simulink model "AUAV_V3_TestSensors"  (R2015a)
settings: Solver=FixedStepDiscrete  StartTime=0.0  StopTime=10.0  FixedStep=T  RelTol=1e-3
PreLoadFcn:
  | %T = 0.0025;
  | MavlinkBus;
  | mcuInit;
  | % Baro Altitude Computation
  | % =========================
  | basePressure = 98192.64;
  | baseTemp = 288.215;
  | lapseRate = -0.00198122;
  | baseHeight = 0;
values from neighbouring files (symbols this model uses):
  apSampleTime = 0.01    [mcuInit.m]
  latlong_WP = 1    [mcuInit.m]
  mavlink_attitude_t = Simulink.Bus    [MavlinkBusMarcello.m]
  mavlink_gps_raw_int_t = Simulink.Bus    [MavlinkBus.m]    (also in MavlinkBusMarcello.m)
  mavlink_raw_imu_t = Simulink.Bus    [MavlinkBus.m]    (also in MavlinkBusMarcello.m)
  mavlink_scaled_pressure_t = Simulink.Bus    [MavlinkBus.m]    (also in MavlinkBusMarcello.m)
  mavlink_servo_output_raw_t = Simulink.Bus    [MavlinkBusMarcello.m]
  mavlink_slugs_navigation_t = Simulink.Bus    [MavlinkBusMarcello.m]
  mavlink_sys_status_t = Simulink.Bus    [MavlinkBus.m]    (also in MavlinkBusMarcello.m)
  T = 0.01    [mcuInit.m]
  Xpoints = [0 0]    [mcuInit.m]
  Ypoints = [0 0]    [mcuInit.m]
  Zpoints = [0 0]    [mcuInit.m]
undefined symbols (not defined in the file or in its folder): A0, A14, A15, A2, A3, A4, A5, A6, accBiasRateLimit, B0, bankCommandLimit, barAdjust, baroCutoff, baroCutTemp, cubeAccelGain16405, cubeGyroGain16405, cubeMagGain16405, D0, D11, D7, D8, daLimit, data, daTrimMax, daTrimMin, deLimit, deTrimMax, deTrimMin, drLimit, drTrimMax, drTrimMin, dtLimit, dtTrimMax, dtTrimMin, F2, F3, G0, G13, G15, gaind, GS_location, gyroBiasRateLimit, IC1max, IPStar, ISA_g, Max, maxAcc, MaxDwnPthStar, maxDynPressure, maxEta, mlParamInterface, ms, OC1max, P112, P125, P127, P16, P20, P21, P30 ... (+26)
undefined symbols (not defined in the file): baroOffset, baroScale, barTGain1, barTGain2, barTMean1, barTMean2, bda, bde, bdr, bdt, bICda, bICde, bICdr, bICdt, derivativesConstant, lowRateSensorCutoff, mainSensorCutoff, mda, mde, mdr, mdt, mICda, mICde, mICdr, mICdt, pitotOffset, pitotScale, pitTGain1, pitTGain2, pitTMean1, pitTMean2, powerOffset, powerScale, pressureSensorCutoff, tempOffset, tempScale, vzCutoff, xCutoff, yCutoff
libraries: MCHP_Blockset x158, simulink x84, SLUGS_Library x31, aerolibconvert2 x6, aerolibutil x4, aerolibtransform2 x3, dspmtrx3 x2, aerolibobsolete x2
(part 13 of 24)

== system AUAV_V3_TestSensors/Inner Loop// Navigation/L1 Output Feedback Controller With Projection Operator/Trapezoidal Integrator ==
  x : Inport
  Reset : Inport  Port=2
  Constant : Constant  Value=1/3  OutDataTypeStr=single
  Constant1 : Constant  Value=4/3  OutDataTypeStr=single
  Constant2 : Constant  Value=T/2  OutDataTypeStr=single
  Constant3 : Constant  Value=1/3  OutDataTypeStr=single
  Constant5 : Constant  Value=0  OutDataTypeStr=single
  Integer Delay : Delay  DelayLength=1  InputProcessing=Inherited  SampleTime=T
  Integer Delay1 : Delay  InputProcessing=Inherited  SampleTime=T
  Integer Delay2 : Delay  DelayLength=1  InputProcessing=Inherited  SampleTime=T
  Product{,1..3} (4 alike) : Product  OutDataTypeStr=single  RndMeth=Zero
  Protect NaNs : Subsystem
  Protect NaNs1 : Subsystem
  Subtract : Sum  Inputs=3  OutDataTypeStr=single
  Subtract1 : Sum  Inputs=2  OutDataTypeStr=single
  Switch1 : Switch  Criteria=u2 > Threshold  Threshold=0.3  SampleTime=.01
  "[min max]" : Saturate  UpperLimit=upperLimit  LowerLimit=lowerLimit  SampleTime=T
  Int(x) : Outport
  wires:
  Constant/1 -> Product/2
  Constant1/1 -> Product1/2
  Integer Delay/1 -> Product1/1
  Integer Delay1/1 -> Product2/1
  Constant3/1 -> Product2/2
  x/1 -> Protect NaNs/1(In1)
  Product/1 -> Subtract/1
  Product1/1 -> Subtract/2
  Product2/1 -> Subtract/3
  Constant2/1 -> Product3/1
  Subtract/1 -> Product3/2
  Integer Delay2/1 -> Subtract1/1
  Constant5/1 -> Switch1/1
  Reset/1 -> Switch1/2
  Switch1/1 -> Protect NaNs1/1(In1)
  "[min max]"/1 -> Switch1/3
  Product3/1 -> Subtract1/2
  Subtract1/1 -> "[min max]"/1
  Protect NaNs/1(Out1) -> Product/1, Integer Delay/1, Integer Delay1/1
  Protect NaNs1/1(Out1) -> Int(x)/1, Integer Delay2/1

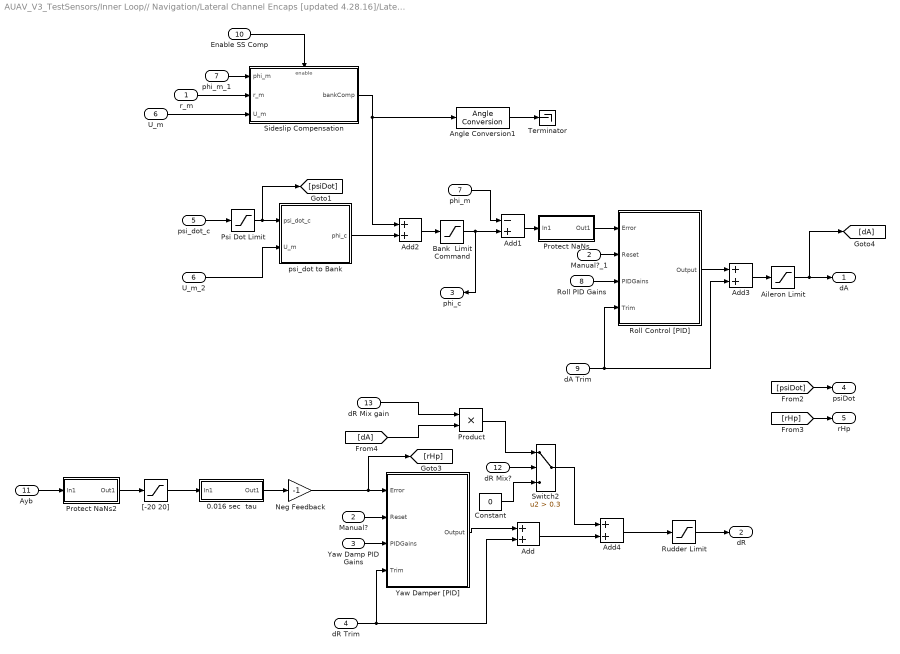
== system AUAV_V3_TestSensors/Inner Loop// Navigation/Lateral Channel Encaps [updated 4.28.16]/Lateral Channel ==
  r_m : Inport
  Manual? : Inport  Port=2
  Yaw Damp PID Gains : Inport  Port=3
  dR Trim : Inport  Port=4
  psi_dot_c : Inport  Port=5
  U_m : Inport  Port=6
  phi_m : Inport  Port=7
  Roll PID Gains : Inport  Port=8
  dA Trim : Inport  Port=9
  Enable SS Comp : Inport  Port=10
  Ayb : Inport  Port=11
  dR Mix? : Inport  Port=12
  dR Mix gain : Inport  Port=13
  0.016 sec  tau : Subsystem  mask(Tustin1stOrderLowpassAutoInitialCondition){f=10, T=T}
      mask prompts: f "Lowpass Frequency"; T "Sample Time"
      mask help: Takes a 3db rolloff frequency (in Hz, NOT radians/s) and a sample time. Performs a symbolic Tustin conversion and implements in a discrete filter. The initial output of the filter is set by the first sample.
      mask Help: Enter the desired 3db rolloff frequency in Hz and the sample time. Initial conditions are sampled automatically.
      mask Display: fprintf('%.2f Hz lowpass',f)
  Add{,2..4} (4 alike) : Sum  OutDataTypeStr=single
  Add1 : Sum  Inputs=-+  OutDataTypeStr=single
  Aileron Limit : Saturate  UpperLimit=daLimit  LowerLimit=-daLimit  SampleTime=apSampleTime
  Angle Conversion1 : aerolibconvert2/Angle Conversion  IU=rad  OU=deg
  Bank  Limit Command : Saturate  UpperLimit=bankCommandLimit  LowerLimit=-bankCommandLimit  SampleTime=apSampleTime
  Constant : Constant  Value=0  OutDataTypeStr=single
  Manual?_1 : InportShadow  Port=2
  "Neg Feedback " : Gain  Gain=-1  OutDataTypeStr=float('single')
  Product : Product  RndMeth=Zero
  Protect NaNs : Subsystem
  Protect NaNs2 : Subsystem
  Psi Dot Limit : Saturate  UpperLimit=1  LowerLimit=-1  SampleTime=apSampleTime
  Roll Control [PID] : Subsystem  AncestorBlock=SLUGS_Library/Control Blocks/PID Controller w//Anti-Windup  mask(PID){Tsample=apSampleTime, Ndelay=derivativesConstant, upperSaturationLimit=daLimit, lowerSaturationLimit=-daLimit}
      mask prompts: Tsample "Sample Time"; Ndelay "Integer delays for de/dt"; upperSaturationLimit "Upper Saturation Limit"; lowerSaturationLimit "Lower Saturation Limit"
      mask help: PID controller block with anti-windup and saturation limits. Implemented as a discrete forwardl integration which stops integrating when the output is saturated. Derivative is implemented as a numerical derivative with N integer delays to smooth output.
      mask Display:
      | disp('PID')
      | port_label('input',1,'error')
      | port_label('input',3,'gains')
      | port_label('input',2,'reset')
      | port_label('input',4,'trim')
      | port_label('output',1,'output')
  Rudder Limit : Saturate  UpperLimit=drLimit  LowerLimit=-drLimit  SampleTime=apSampleTime
  Sideslip Compensation : Subsystem
  Switch2 : Switch  Criteria=u2 > Threshold  Threshold=0.3  InputSameDT=on
  Terminator : Terminator
  U_m_2 : InportShadow  Port=6
  Yaw Damper [PID] : Subsystem  AncestorBlock=SLUGS_Library/Control Blocks/PID Controller w//Anti-Windup  mask(PID){Tsample=apSampleTime, Ndelay=derivativesConstant, upperSaturationLimit=drLimit, lowerSaturationLimit=-drLimit}
      mask prompts: Tsample "Sample Time"; Ndelay "Integer delays for de/dt"; upperSaturationLimit "Upper Saturation Limit"; lowerSaturationLimit "Lower Saturation Limit"
      mask help: PID controller block with anti-windup and saturation limits. Implemented as a discrete forwardl integration which stops integrating when the output is saturated. Derivative is implemented as a numerical derivative with N integer delays to smooth output.
      mask Display:
      | disp('PID')
      | port_label('input',1,'error')
      | port_label('input',3,'gains')
      | port_label('input',2,'reset')
      | port_label('input',4,'trim')
      | port_label('output',1,'output')
  "[-20 20]" : Saturate  UpperLimit=20  LowerLimit=-20
  phi_m_1 : InportShadow  Port=7
  psi_dot to Bank : Subsystem  AncestorBlock=SLUGS_Library/Navigation/psi_dot to Bank
  dA : Outport
  dR : Outport  Port=2
  phi_c : Outport  Port=3
  psiDot : Outport  Port=4
  rHp : Outport  Port=5
  wires:
  [rHp] -> rHp/1
  [psiDot] -> psiDot/1
  [dA] -> Product/2
  dR Mix gain/1 -> Product/1
  Product/1 -> Switch2/1
  Constant/1 -> Switch2/3
  dR Mix?/1 -> Switch2/2
  Switch2/1 -> Add4/1
  Add/1 -> Add4/2
  Add4/1 -> Rudder Limit/1
  Angle Conversion1/1 -> Terminator/1
  "[-20 20]"/1 -> 0.016 sec  tau/1(In1)
  Protect NaNs2/1(Out1) -> "[-20 20]"/1
  Protect NaNs/1(Out1) -> Roll Control [PID]/1(Error)
  Rudder Limit/1 -> dR/1
  0.016 sec  tau/1(Out1) -> "Neg Feedback "/1
  "Neg Feedback "/1 -> Yaw Damper [PID]/1(Error), [rHp]
  Ayb/1 -> Protect NaNs2/1(In1)
  Enable SS Comp/1 -> Sideslip Compensation/Enable
  U_m/1 -> Sideslip Compensation/3(U_m)
  r_m/1 -> Sideslip Compensation/2(r_m)
  phi_m_1/1 -> Sideslip Compensation/1(phi_m)
  Sideslip Compensation/1(bankComp) -> Angle Conversion1/1, Add2/1
  psi_dot to Bank/1(phi_c) -> Add2/2
  Add2/1 -> Bank  Limit Command/1
  U_m_2/1 -> psi_dot to Bank/2(U_m)
  Manual?/1 -> Yaw Damper [PID]/2(Reset)
  Yaw Damp PID Gains/1 -> Yaw Damper [PID]/3(PIDGains)
  Yaw Damper [PID]/1(Output) -> Add/1
  dR Trim/1 -> Yaw Damper [PID]/4(Trim), Add/2
  Manual?_1/1 -> Roll Control [PID]/2(Reset)
  Roll PID Gains/1 -> Roll Control [PID]/3(PIDGains)
  Add3/1 -> Aileron Limit/1
  Roll Control [PID]/1(Output) -> Add3/1
  dA Trim/1 -> Roll Control [PID]/4(Trim), Add3/2
  Aileron Limit/1 -> [dA], dA/1
  Add1/1 -> Protect NaNs/1(In1)
  phi_m/1 -> Add1/1
  Bank  Limit Command/1 -> phi_c/1, Add1/2
  Psi Dot Limit/1 -> [psiDot], psi_dot to Bank/1(psi_dot_c)
  psi_dot_c/1 -> Psi Dot Limit/1

== system AUAV_V3_TestSensors/Inner Loop// Navigation/Lateral Channel Encaps [updated 4.28.16]/psi_dot_c Select logic1 ==
  psi_dot_ad : Inport
  L1OnOff : Inport  Port=2
  psi_dot_c_noNav : Inport  Port=3
  IsPassThrough : Inport  Port=4
  nav_phi_c : Inport  Port=5
  U_m : Inport  Port=6
  Bank to Psi Dot : Subsystem  AncestorBlock=SLUGS_Library/Navigation/Bank to Psi Dot
  Switch : Switch  Criteria=u2 > Threshold  Threshold=0.3
  Switch1 : Switch  Criteria=u2 > Threshold  Threshold=0.3  InputSameDT=on
  psi_dot_c : Outport
  psi_dot_c_4_L1 : Outport  Port=2
  wires:
  U_m/1 -> Bank to Psi Dot/2(U_m)
  nav_phi_c/1 -> Bank to Psi Dot/1(phi_c)
  IsPassThrough/1 -> Switch1/2
  psi_dot_c_noNav/1 -> Switch1/1
  Switch/1 -> psi_dot_c/1
  L1OnOff/1 -> Switch/2
  psi_dot_ad/1 -> Switch/1
  Switch1/1 -> psi_dot_c_4_L1/1, Switch/3
  Bank to Psi Dot/1(psi_dot_c) -> Switch1/3

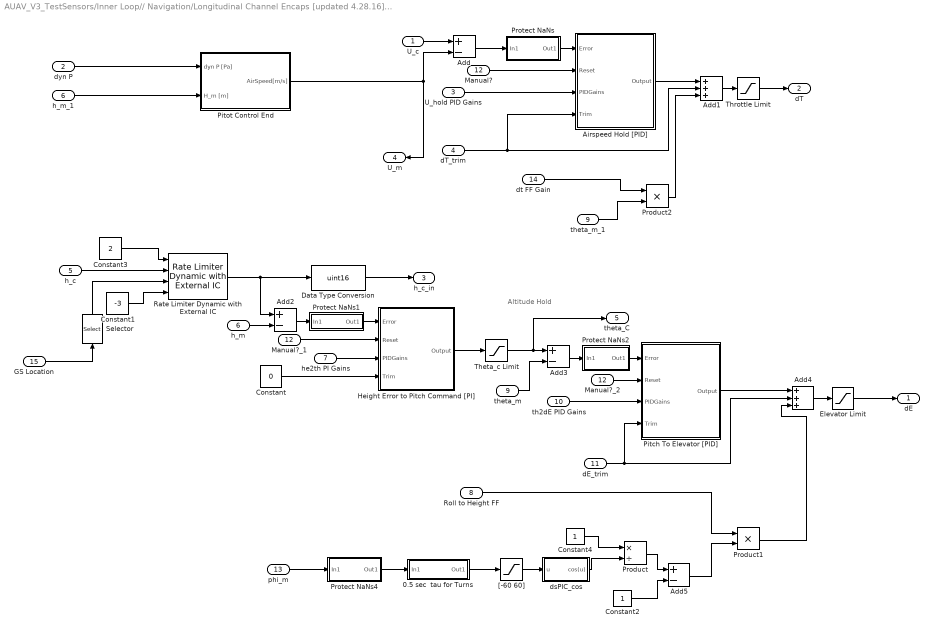
== system AUAV_V3_TestSensors/Inner Loop// Navigation/Longitudinal Channel Encaps [updated 4.28.16]/Longitudinal Channel ==
  note: Altitude Hold
  U_c : Inport
  dyn P : Inport  Port=2
  U_hold PID Gains : Inport  Port=3
  dT_trim : Inport  Port=4
  h_c : Inport  Port=5
  h_m : Inport  Port=6
  he2th PI Gains : Inport  Port=7
  Roll to Height FF : Inport  Port=8
  theta_m : Inport  Port=9
  th2dE PID Gains : Inport  Port=10
  dE_trim : Inport  Port=11
  Manual? : Inport  Port=12
  phi_m : Inport  Port=13
  dt FF Gain : Inport  Port=14
  GS Location : Inport  Port=15
  0.5 sec  tau for Turns : Subsystem  mask(Tustin1stOrderLowpassAutoInitialCondition){f=0.32, T=T}
      mask prompts: f "Lowpass Frequency"; T "Sample Time"
      mask help: Takes a 3db rolloff frequency (in Hz, NOT radians/s) and a sample time. Performs a symbolic Tustin conversion and implements in a discrete filter. The initial output of the filter is set by the first sample.
      mask Help: Enter the desired 3db rolloff frequency in Hz and the sample time. Initial conditions are sampled automatically.
      mask Display: fprintf('%.2f Hz lowpass',f)
  Add : Sum  Inputs=+-
  Add1 : Sum  Inputs=3  OutDataTypeStr=single
  Add2 : Sum  Inputs=+-  OutDataTypeStr=single
  Add3 : Sum  Inputs=+-  OutDataTypeStr=single
  Add4 : Sum  Inputs=3  OutDataTypeStr=single
  Add5 : Sum  Inputs=+-  OutDataTypeStr=single
  Airspeed Hold [PID] : Subsystem  AncestorBlock=SLUGS_Library/Control Blocks/PID Controller w//Anti-Windup  mask(PID){Tsample=apSampleTime, Ndelay=derivativesConstant, upperSaturationLimit=dtLimit, lowerSaturationLimit=0}
      mask prompts: Tsample "Sample Time"; Ndelay "Integer delays for de/dt"; upperSaturationLimit "Upper Saturation Limit"; lowerSaturationLimit "Lower Saturation Limit"
      mask help: PID controller block with anti-windup and saturation limits. Implemented as a discrete forwardl integration which stops integrating when the output is saturated. Derivative is implemented as a numerical derivative with N integer delays to smooth output.
      mask Display:
      | disp('PID')
      | port_label('input',1,'error')
      | port_label('input',3,'gains')
      | port_label('input',2,'reset')
      | port_label('input',4,'trim')
      | port_label('output',1,'output')
  Constant : Constant  Value=0
  Constant1 : Constant  Value=-3  OutDataTypeStr=single
  Constant2 : Constant  OutDataTypeStr=single
  Constant3 : Constant  Value=2  OutDataTypeStr=single
  Constant4 : Constant  OutDataTypeStr=single
  Data Type Conversion : DataTypeConversion  OutDataTypeStr=uint16
  Elevator Limit : Saturate  UpperLimit=deLimit  LowerLimit=-deLimit  SampleTime=apSampleTime
  Height Error to Pitch Command [PI] : Subsystem  AncestorBlock=SLUGS_Library/Control Blocks/PI Controller w//Anti-Windup  mask(PID){Tsample=apSampleTime, Ndelay=derivativesConstant, upperSaturationLimit=pitchCommandLimit, lowerSaturationLimit=-pitchCommandLimit}
      mask prompts: Tsample "Sample Time"; Ndelay "Integer delays for de/dt"; upperSaturationLimit "Upper Saturation Limit"; lowerSaturationLimit "Lower Saturation Limit"
      mask help: PID controller block with anti-windup and saturation limits. Implemented as a discrete forwardl integration which stops integrating when the output is saturated. Derivative is implemented as a numerical derivative with N integer delays to smooth output.
      mask Display:
      | disp('PI')
      | port_label('input',1,'error')
      | port_label('input',3,'gains')
      | port_label('input',2,'reset')
      | port_label('input',4,'trim')
      | port_label('output',1,'output')
  Manual?_1 : InportShadow  Port=12
  Manual?_2 : InportShadow  Port=12
  Pitch To Elevator [PID] : Subsystem  AncestorBlock=SLUGS_Library/Control Blocks/PID Controller w//Anti-Windup  mask(PID){Tsample=apSampleTime, Ndelay=derivativesConstant, upperSaturationLimit=deLimit, lowerSaturationLimit=-deLimit}
      mask prompts: Tsample "Sample Time"; Ndelay "Integer delays for de/dt"; upperSaturationLimit "Upper Saturation Limit"; lowerSaturationLimit "Lower Saturation Limit"
      mask help: PID controller block with anti-windup and saturation limits. Implemented as a discrete forwardl integration which stops integrating when the output is saturated. Derivative is implemented as a numerical derivative with N integer delays to smooth output.
      mask Display:
      | disp('PID')
      | port_label('input',1,'error')
      | port_label('input',3,'gains')
      | port_label('input',2,'reset')
      | port_label('input',4,'trim')
      | port_label('output',1,'output')
  Pitot Control End : Subsystem  AncestorBlock=SLUGS_Library/Sensor Blocks/Pitot Control End
  Product : Product  Inputs=*/  RndMeth=Zero
  Product1 : Product  RndMeth=Zero
  Product2 : Product  RndMeth=Zero
  Protect NaNs : Subsystem
  Protect NaNs1 : Subsystem
  Protect NaNs2 : Subsystem
  Protect NaNs4 : Subsystem
  Rate Limiter Dynamic with External IC : SLUGS_Library/Singnal Routing & Conditioning/Rate Limiter Dynamic with External IC  rlIC=0
  Selector : Selector  InputPortWidth=3  Indices=[1 ]
  Theta_c Limit : Saturate  UpperLimit=pitchCommandLimit  LowerLimit=-pitchCommandLimit  SampleTime=apSampleTime
  Throttle Limit : Saturate  UpperLimit=dtLimit  LowerLimit=0  SampleTime=apSampleTime
  "[-60 60]" : Saturate  UpperLimit=60  LowerLimit=-60  SampleTime=apSampleTime
  dsPIC_cos : Subsystem  AncestorBlock=SLUGS_Library/dsPIC_cos
  h_m_1 : InportShadow  Port=6
  theta_m_1 : InportShadow  Port=9
  dE : Outport
  dT : Outport  Port=2
  h_c_in : Outport  Port=3
  U_m : Outport  Port=4
  theta_C : Outport  Port=5
  wires:
  GS Location/1 -> Selector/1
  Protect NaNs4/1(Out1) -> 0.5 sec  tau for Turns/1(In1)
  Protect NaNs2/1(Out1) -> Pitch To Elevator [PID]/1(Error)
  Protect NaNs1/1(Out1) -> Height Error to Pitch Command [PI]/1(Error)
  Protect NaNs/1(Out1) -> Airspeed Hold [PID]/1(Error)
  Constant/1 -> Height Error to Pitch Command [PI]/4(Trim)
  U_hold PID Gains/1 -> Airspeed Hold [PID]/3(PIDGains)
  dt FF Gain/1 -> Product2/1
  Product2/1 -> Add1/3
  theta_m_1/1 -> Product2/2
  Product1/1 -> Add4/3
  Roll to Height FF/1 -> Product1/1
  Add5/1 -> Product1/2
  "[-60 60]"/1 -> dsPIC_cos/1(u)
  0.5 sec  tau for Turns/1(Out1) -> "[-60 60]"/1
  Product/1 -> Add5/1
  Constant4/1 -> Product/1
  dsPIC_cos/1(cos(u)) -> Product/2
  Constant2/1 -> Add5/2
  phi_m/1 -> Protect NaNs4/1(In1)
  Pitot Control End/1(AirSpeed[m/s]) -> U_m/1, Add/2
  U_c/1 -> Add/1
  Add/1 -> Protect NaNs/1(In1)
  Airspeed Hold [PID]/1(Output) -> Add1/1
  dT_trim/1 -> Airspeed Hold [PID]/4(Trim), Add1/2
  Add1/1 -> Throttle Limit/1
  Throttle Limit/1 -> dT/1
  Add2/1 -> Protect NaNs1/1(In1)
  h_m/1 -> Add2/2
  theta_m/1 -> Add3/2
  Manual?/1 -> Airspeed Hold [PID]/2(Reset)
  Manual?_1/1 -> Height Error to Pitch Command [PI]/2(Reset)
  Manual?_2/1 -> Pitch To Elevator [PID]/2(Reset)
  Add4/1 -> Elevator Limit/1
  Pitch To Elevator [PID]/1(Output) -> Add4/1
  dE_trim/1 -> Pitch To Elevator [PID]/4(Trim), Add4/2
  Elevator Limit/1 -> dE/1
  dyn P/1 -> Pitot Control End/1(dyn P [Pa])
  h_m_1/1 -> Pitot Control End/2(H_m [m])
  he2th PI Gains/1 -> Height Error to Pitch Command [PI]/3(PIDGains)
  th2dE PID Gains/1 -> Pitch To Elevator [PID]/3(PIDGains)
  Add3/1 -> Protect NaNs2/1(In1)
  Theta_c Limit/1 -> theta_C/1, Add3/1
  Rate Limiter Dynamic with External IC/1 -> Data Type Conversion/1, Add2/1
  Height Error to Pitch Command [PI]/1(Output) -> Theta_c Limit/1
  Constant3/1 -> Rate Limiter Dynamic with External IC/1
  Selector/1 -> Rate Limiter Dynamic with External IC/3
  Constant1/1 -> Rate Limiter Dynamic with External IC/4
  h_c/1 -> Rate Limiter Dynamic with External IC/2
  Data Type Conversion/1 -> h_c_in/1

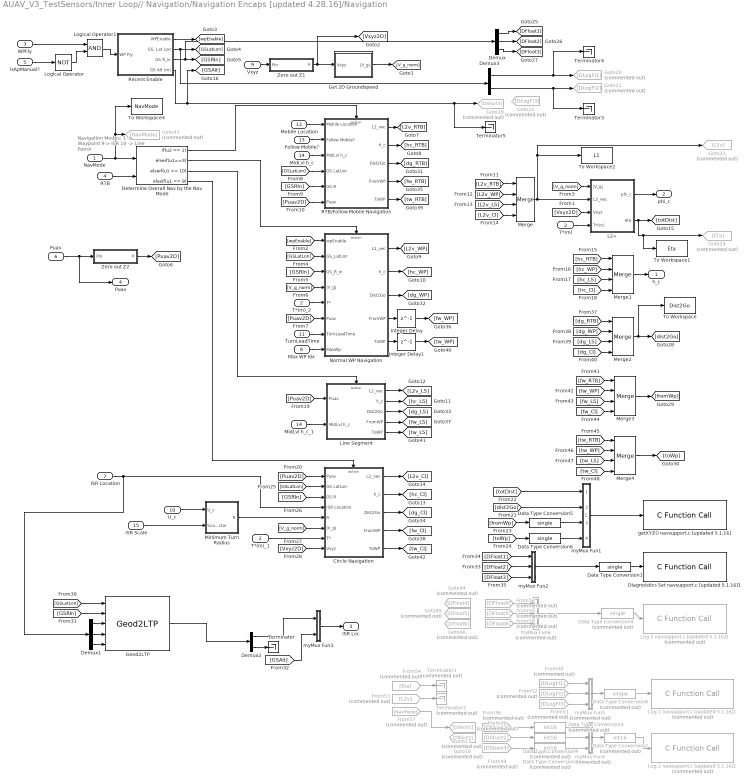
== system AUAV_V3_TestSensors/Inner Loop// Navigation/Navigation Encaps [updated 4.28.16]/Navigation ==
  note: Navigation Modes:
      | 3 -> Waypoint
      | 9-> ISR
      | 10 -> Line Patrol
  NavMode : Inport
  T*(m) : Inport  Port=2
  WPFly : Inport  Port=3
  RTB : Inport  Port=4
  isApManual? : Inport  Port=5
  Puav : Inport  Port=6  SampleTime=apSampleTime
  ISR Location : Inport  Port=7
  Max WP Idx : Inport  Port=8
  Vxyz : Inport  Port=9  SampleTime=apSampleTime
  U_c : Inport  Port=10
  TurnLeadTime : Inport  Port=11
  Mobile Location : Inport  Port=12
  Follow Mobile? : Inport  Port=13
  MidLvl h_c : Inport  Port=14
  ISR Scale : Inport  Port=15
  Circle Navigation : Subsystem  TreatAsAtomicUnit=on
  Data Type Conversion1 : DataTypeConversion  OutDataTypeStr=single
  Data Type Conversion{2..4,7} (4 alike) : DataTypeConversion  Commented=on  OutDataTypeStr=int16
  Data Type Conversion5 : DataTypeConversion  OutDataTypeStr=single
  Data Type Conversion6 : DataTypeConversion  OutDataTypeStr=single
  Data Type Conversion8 : DataTypeConversion  Commented=on  OutDataTypeStr=single
  Data Type Conversion9 : DataTypeConversion  Commented=on  OutDataTypeStr=single
  Demux : Demux  Outputs=3
  Demux1 : Demux  Outputs=3
  Demux2 : Demux  Outputs=[2 1]
  Demux3 : Demux  Outputs=2
  Determine Overall Nav by the Nav Mode : If  NumInputs=2  IfExpression=u2 == 1  ElseIfExpressions=u1==3, u1 == 10, u1 == 9  ShowElse=off
  Diagnoistics Set navsupport.c [updated 5.1.16]1 : MCHP_Blockset/User Functions/C Function Call  ParseFilesChkbx=off  ListFunctions1=Custom Function  Function1=void setDiagnosticFloat(float * flValues)  AddHeaderDeclaration=on  Function1Type=when block is updated (default)  Fct1BlockIn=flValues  FctReturnBlockOut=on  DataCollected=0  ORDERING=None  SampleTime=-1  MCHP_MASTERLINK=|  PinDigitalInput=[]  PinDigitalOutput=[]  PinAnalogInput=[]
      | AUAV_V3_TestSensors/Microchip Master
      | AUAV V3 Board
      | Busy Flag on D2 (RA6)
  From29 : From  Commented=on  GotoTag=DShort2
  From36 : From  Commented=on  GotoTag=DShort1
  From49 : From  Commented=on  GotoTag=DShort3
  From50 : From  Commented=on  GotoTag=DLogFl1
  From51 : From  Commented=on  GotoTag=DLogFl3
  From52 : From  Commented=on  GotoTag=DLogFl2
  From53 : From  Commented=on  GotoTag=L2v
  From54 : From  Commented=on  GotoTag=Eta
  From55 : From  Commented=on  GotoTag=DFloat5
  From56 : From  Commented=on  GotoTag=DFloat4
  From57 : From  Commented=on  GotoTag=NavMode
  From58 : From  Commented=on  GotoTag=DFloat6
  Geod2LTP : SLUGS_Library/Navigation/Geod2LTP
  Get 2D Groundspeed : Subsystem
  Goto17 : Goto  Commented=on  GotoTag=DShort1
  Goto18 : Goto  Commented=on  GotoTag=DShort2
  Goto19 : Goto  Commented=on  GotoTag=DShort3
  Goto20 : Goto  Commented=on  GotoTag=DLogFl1
  Goto21 : Goto  Commented=on  GotoTag=DLogFl2
  Goto22 : Goto  Commented=on  GotoTag=DLogFl3
  Goto23 : Goto  Commented=on  GotoTag=L2v
  Goto24 : Goto  Commented=on  GotoTag=Eta
  Goto43 : Goto  Commented=on  GotoTag=NavMode
  Goto44 : Goto  Commented=on  GotoTag=DFloat4
  Goto45 : Goto  Commented=on  GotoTag=DFloat5
  Goto46 : Goto  Commented=on  GotoTag=DFloat6
  Integer Delay : Delay  DelayLength=1  InputProcessing=Inherited
  Integer Delay1 : Delay  DelayLength=1  InputProcessing=Inherited
  L2+ : Subsystem
  Line Segment : Subsystem  TreatAsAtomicUnit=on
  Log 1 navsupport.c [updated 5.1.16]1 : MCHP_Blockset/User Functions/C Function Call  Commented=on  ParseFilesChkbx=off  ListFunctions1=Custom Function  Function1=void setDiagnosticFloat(float * flValues)  AddHeaderDeclaration=on  Function1Type=when block is updated (default)  Fct1BlockIn=flValues  FctReturnBlockOut=on  DataCollected=0  ORDERING=None  SampleTime=-1  MCHP_MASTERLINK=|  PinDigitalInput=[]  PinDigitalOutput=[]  PinAnalogInput=[]
      | AUAV_V3_TestSensors/Microchip Master
      | AUAV V3 Board
      | Busy Flag on D2 (RA6)
  Log 2 navsupport.c [updated 5.1.16]1 : MCHP_Blockset/User Functions/C Function Call  Commented=on  ParseFilesChkbx=off  ListFunctions1=Custom Function  Function1=void setDiagnosticShort(int16_t *shValues)  AddHeaderDeclaration=on  Function1Type=when block is updated (default)  Fct1BlockIn=shValues  FctReturnBlockOut=on  DataCollected=0  ORDERING=None  SampleTime=-1  MCHP_MASTERLINK=|  PinDigitalInput=[]  PinDigitalOutput=[]  PinAnalogInput=[]
      | AUAV_V3_TestSensors/Microchip Master
      | AUAV V3 Board
      | Busy Flag on D2 (RA6)
  Log 2 navsupport.c [updated 5.1.16]2 : MCHP_Blockset/User Functions/C Function Call  Commented=on  ParseFilesChkbx=off  ListFunctions1=Custom Function  Function1=void setDiagnosticFloat(float * flValues)  AddHeaderDeclaration=on  Function1Type=when block is updated (default)  Fct1BlockIn=flValues  FctReturnBlockOut=on  DataCollected=0  ORDERING=None  SampleTime=-1  MCHP_MASTERLINK=|  PinDigitalInput=[]  PinDigitalOutput=[]  PinAnalogInput=[]
      | AUAV_V3_TestSensors/Microchip Master
      | AUAV V3 Board
      | Busy Flag on D2 (RA6)
  Logical Operator : Logic  Operator=NOT  AllPortsSameDT=off  OutDataTypeStr=boolean
  Logical Operator1 : Logic  AllPortsSameDT=off  OutDataTypeStr=boolean
  Merge{,1..4} (5 alike) : Merge  Inputs=4
  MidLvl h_c_1 : InportShadow  Port=14
  Minimum Turn Radius : Subsystem
  Normal WP Navigation : Subsystem  TreatAsAtomicUnit=on
  RTB/Follow Mobile Navigation : Subsystem
  Recent Enable : Subsystem
  T*(m)_1 : InportShadow  Port=2
  T*(m)_2 : InportShadow  Port=2
  Terminator{,3..5} (4 alike) : Terminator
  Terminator1 : Terminator  Commented=on
  Terminator2 : Terminator  Commented=on
  To Workspace : ToWorkspace  VariableName=Dist2Go  SampleTime=-1
  To Workspace1 : ToWorkspace  VariableName=Eta  SampleTime=-1
  To Workspace2 : ToWorkspace  VariableName=L1  SampleTime=-1
  To Workspace4 : ToWorkspace  VariableName=NavMode  SampleTime=-1
  Zero out Z1 : MATLAB Function  TreatAsAtomicUnit=on
  Zero out Z2 : MATLAB Function  TreatAsAtomicUnit=on
  getXYZ() navsupport.c [updated 5.1.16] : MCHP_Blockset/User Functions/C Function Call  ParseFilesChkbx=on  ListFunctions1=Custom Function  Function1=void setNavNav(float* values)  AddHeaderDeclaration=on  Function1Type=when block is updated (default)  Fct1BlockIn=values  FctReturnBlockOut=on  DataCollected="s.chksm=reshape({ '638529-אוק-2016 01:00:36','251929-אוק-2016 01:00:36','1689429-אוק-2016 01:00:36','4250714-אוק-2016 08:45:05','360329-אוק-2016 01:00:36','7293729-אוק-2016 01:00:36','954929-אוק-2016 01:00:36','296129-אוק-2016 01:00:36','278129-אוק-2016 01:00:36','556029-אוק-2016 01:00:36','963229-אוק-2016 01:00:36','1122729-אוק-2016 01:00:36','372429-אוק-2016 01:00:36','998829-אוק-2016 01:00:36','536514-אוק-2016 08:45:05'},1,15);s.File1=reshape({ '  void  newCircBuffer(CBRef cB)','  void  freeCircBuffer(CBRef* cB)','  void  freeCircBuffer(CBRef* cB)',' unsigned int  getLength(CBRef cB)','  int  readHead(CBRef cB)','  int  readTail(CBRef cB)',' unsigned char  peak(CBRef cB)',' unsigned char  readFront(CBRef cB)',' unsigned char  writeBack(CBRef cB, unsigned char data)','  void  makeEmpty(CBRef cB)','  void  printCircBuf(CBRef cB)'},1,11);s.File2=reshape({ '  void  uartBufferInit(void)','  void  __attribute__((__interrupt__, no_auto_psv)) _U4RXInterrupt(void)','  void  getGPSRawData(unsigned char* gpsBuffer)',' unsigned char  isGPSNovatel(void)'},1,4);s.File3=reshape({ '  char  hex2char(char halfhex)','  float  degMinToDeg(unsigned char degrees, float minutes)',' unsigned char  gpsUbloxSeparate(unsigned char* outStream)','  void  gpsUbloxParse(void)','  void  getGpsUbloxMainData(float* data)','  void  getGpsUbloxData(float* data)','  char  gpSmbl(char symbl)',' unsigned char  myTokenizer(char* stringToTokenize, char token, char * returnToken)','  void  parseRMC(unsigned char* stream)','  void  parseGGA(unsigned char* stream)',' unsigned char  getChecksum(unsigned char* sentence, unsigned char size)','  void  gpsDebugMsg(unsigned char buf)'},1,12);s.File4=reshape({ '  void  uartMavlinkBufferInit(void)','  void __attribute__((__interrupt__,__auto_psv__)) _U1RXInterrupt(void)','  uint8_t  isFinite(float s)','  void  InitParameterInterface(void)','  void  protDecodeMavlink(void)','  uint16_t  MissionInterfaceResponse(uint8_t system_id, uint8_t component_id)','  uint16_t  ParameterInterfaceResponse(uint8_t system_id, uint8_t component_id)','  uint16_t  PackHeartBeat(uint8_t system_id, uint8_t component_id)','  uint16_t  PackTextMsg(uint8_t system_id, uint8_t component_id, unsigned char buf)','  uint16_t  PackRawIMU(uint8_t system_id, uint8_t component_id, mavlink_raw_imu_t mlRawIMUData ,uint32_t time_usec)','  uint16_t  PackRawAttitude(uint8_t system_id, uint8_t component_id, mavlink_attitude_t mlAttitudeData ,uint32_t time_usec)','  uint16_t  PackPosXYZ_Sol(uint8_t system_id, uint8_t component_id, mavlink_local_position_ned_t mlLocalPositionSol ,uint32_t time_usec)','  uint16_t  PackGpsRawInt(uint8_t system_id, uint8_t component_id, mavlink_gps_raw_int_t mlRawGpsDataInt ,uint32_t time_usec)','  uint16_t  PackScaledPressure(uint8_t system_id, uint8_t component_id, mavlink_scaled_pressure_t mlAirData ,uint32_t time_usec)','  uint16_t  PackSysStatus(uint8_t system_id, uint8_t component_id, mavlink_sys_status_t mlSysStatus)','  uint16_t  PackRawServo(uint8_t system_id, uint8_t component_id, mavlink_servo_output_raw_t mlPwmCommands ,uint32_t time_usec)','  uint16_t  HIL_PackRawServo(uint8_t system_id, uint8_t component_id, mavlink_servo_output_raw_t mlPwmCommands ,uint32_t time_usec)','  uint16_t  PackRawRC(uint8_t system_id, uint8_t component_id, mavlink_rc_channels_raw_t mlRC_Commands ,uint32_t time_usec)','  uint16_t  PackVFR_HUD(uint8_t system_id, uint8_t component_id, mavlink_vfr_hud_t mlVfr_hud ,uint32_t time_usec)','  char  sendQGCDebugMessage(const char * dbgMessage, char severity, unsigned char* bytesToAdd, char positionStart)','  void  TxN_Data_OverU1(uint16_t N)','  void  TxN_Data_OverU4(uint16_t N)'},1,22);s.File5=reshape({ '  float  myAtan2(float num, float denom)','  float  myPow(float x, float toTheN)','  float  mySqrt(float x)','  float  myAbs(float x)','  float  myAtan(float x)','  float  myAsin(float x)','  float  mySin(float x)','  float  myCos(float x)','  float  myTan(float x)','  float  myAcos(float x)','  float  myExp(float x)','  void  hugeDelay(void)','  void  smallDelay(void)','  void  tinyDelay(void)','  void  printToUart2(const char *fmt, ...)'},1,15);s.File6=reshape({ '  void  sendTelemetryMavlink(unsigned char* dataOut)','  void  uart2Init(void)','  void  gsRead(unsigned char* gsChunk)','  void  prepareTelemetryMavlink(unsigned char* dataOut)','  void  prepareTelemetryMavlink(unsigned char* dataOut)','  void  sendTelemetryMavlink(unsigned char* dataOut)','  void  copyBufferToDMA1(unsigned char size)','  void  send2GS(unsigned char* protData)','  uint8_t  clearWaypointsFrom(uint8_t startingWp)','  void  addMessageToSpiOut(mavlink_message_t* msg)'},1,10);s.File7={ '  void  populateParameterInterface(void)'};s.File8={ '  void  mavlinkInit(void)'};s.File9=reshape({ '  void  updatePWM(unsigned short * PWMData)','  void  updatePWMTrim(unsigned short PWMData, unsigned char channel)','  void  updateLoad(uint8_t mcuLoad)','  void  updateEuler(float* newEuler)','  void  updatePQR(float* newPQR)',' unsigned char  getHilOnOff(void)','  uint8_t  getLightsOnOff(void)','  uint8_t  getLightsDayNight(void)','  void  updateVISensor(uint16_t* data)','  void  updatePTZ(int16_t* ptz)'},1,10);s.File10=reshape({ '  void  updateRawADCData(int16_t* adcData)','  void  updateAirData(float* airData)','  void  updateLoadData(uint8_t load, uint16_t mvPower)','  void  updateAttitude(float * attitudeData)','  void  getGSLocation(float* altLatLon)','  void  updateTimeStamp(uint32_t timeSt)','  void  updatePosition(float * posData)','  void  updatePilotConsole(uint16_t * pilData)','  void  updateDiagnosticFl(float* diagFl)','  void  updateDiagnosticSh(int16_t* diagSh)','  void  updateBias(float * biasData)','  void  updateSensorData(float* sens)','  uint8_t  isFixValid(void)','  void  updateSensorDiag(float* diag)'},1,14);s.File11=reshape({ '  void  gpsInit(void)','  void  gpsParse(uint8_t* dataStream)','  void  updateStatus(uint8_t* completeMessage)','  void  updatePositionData(uint8_t* completeMessage)','  void  updateVelocityData(uint8_t* completeMessage)','  void  updateTimeData(uint8_t* completeMessage)','  void  getGpsMainData(float* data)','  uint32_t  CRC32Value(int32_t i)','  uint32_t  CalculateBlockCRC32(uint32_t ulCount, uint8_t *ucBuffer)','  uint16_t  charsToUint16(uint8_t* data)','  uint32_t  charsToUint32(uint8_t* data)','  float  charsToFloat(uint8_t* data)','  double  charsToDouble(uint8_t* data)'},1,13);s.File12=reshape({ '  void  getMidLevelCommands(float* commands)',' unsigned char  isApManual(uint16_t failsafe)','  float  getParamIdx(unsigned char idx)','  void  getRangeOfParams(uint8_t startIdx, uint8_t endIdx, float* parameters)','  float  getDynamic(void)','  void  getAttitude(float* attitude)','  void  getXYZ(float* xyz)','  void  getVned(float* xyz)','  uint8_t  getMaxWp(void)',' unsigned char  isWpFly(void)',' unsigned char  isPassthrough(void)','  void  setDiagnosticFloat(float * flValues)','  void  setDiagnosticShort(int16_t* shValues)','  void  getWP(unsigned char idx, float* WPpos)','  void  setLogFloat1(float * flValues)','  void  setLogFloat2(float * flValues)',' unsigned char  getApControlType(void)',' unsigned char  getPassValues(uint8_t* pasVals)','  void  setCurrentCommands(float airSpeed)','  void  getCurrentGPSPos(float* latLonAlt)','  void  setNavLong(float* values)','  void  setNavLat(float* values)','  void  setNavNav(float* values)','  void  getAccels(float * accels)','  void  getAccBias(float * bias)','  void  getRTB(uint8_t* rtb)','  void  getMobileLocation(float* loc)','  uint8_t  getNavMode(void)','  void  getISRLocation(float* loc)','  uint8_t  getISRCameraOption1(void)',' unsigned short  meanFilter5(unsigned short * values)','  uint8_t  justEnabled(uint8_t enableValue, uint8_t index)',' unsigned char  quickSort(unsigned short *arr, char elements)'},1,33);s.File13=reshape({ '  void  hilRead(unsigned char* hilChunk)','  void  hil_getRawRead(short * rawData)','  void  hil_getVned(float* vned)','  void  hil_getEuler(float* euler)','  void  hil_getRates(float* pqr)','  void  hil_getXYZ(float* xyz)',' unsigned int  hil_getTs(void)','  void  protDecodeHil(uint8_t* dataIn)'},1,8);s.File14=reshape({ '  void  cubeInit(void)','  void  getCubeData(short * cubeData)','  void  updateCubeData(void)','  int16_t  averageData(int16_t* theData, uint8_t count)',' unsigned short  write2Cube(unsigned short data2Send)','  short  convert14BitToShort(short wordData)','  short  convert12BitToShort(short wordData)',' unsigned char  isCube16405(void)'},1,8);s.File15=reshape({ '  void  uartMavlinkBufferInit(void)','  uint16_t  PackHeartBeat(uint8_t system_id, uint8_t component_id)','  uint16_t  PackRawServo(uint8_t system_id, uint8_t component_id, mavlink_servo_output_raw_t mlPwmCommands ,uint32_t time_usec)','  uint16_t  HIL_PackRawServo(uint8_t system_id, uint8_t component_id, mavlink_servo_output_raw_t mlPwmCommands ,uint32_t time_usec)','  uint16_t  PackRawRC(uint8_t system_id, uint8_t component_id, mavlink_rc_channels_raw_t mlRC_Commands, uint32_t time_usec)','  uint16_t  PackVFR_HUD(uint8_t system_id, uint8_t component_id, mavlink_vfr_hud_t mlVfr_hud, uint32_t time_usec)','  uint16_t  PackRawIMU(uint8_t system_id, uint8_t component_id, mavlink_raw_imu_t mlRawIMUData ,uint32_t time_usec)','  uint16_t  PackRawAttitude(uint8_t system_id, uint8_t component_id, mavlink_attitude_t mlAttitudeData ,uint32_t time_usec)','  uint16_t  PackPosXYZ_Sol(uint8_t system_id, uint8_t component_id, mavlink_local_position_ned_t mlLocalPositionSol ,uint32_t time_usec)','  char  sendQGCDebugMessage(const char * dbgMessage, char severity, unsigned char* bytesToAdd, char positionStart)','  uint16_t  PackGpsRawInt(uint8_t system_id, uint8_t component_id, mavlink_gps_raw_int_t mlRawGpsDataInt, uint32_t time_usec)','  uint16_t  PackScaledPressure(uint8_t system_id, uint8_t component_id, mavlink_scaled_pressure_t mlAirData, uint32_t time_usec)','  uint16_t  PackSysStatus(uint8_t system_id, uint8_t component_id, mavlink_sys_status_t mlSysStatus)'},1,13);"  ORDERING=None  SampleTime=-1  MCHP_MASTERLINK=|  PinDigitalInput=[]  PinDigitalOutput=[]  PinAnalogInput=[]
      | AUAV_V3_TestSensors/Microchip Master
      | AUAV V3 Board
      | Busy Flag on D2 (RA6)
  myMux Fun1 : MATLAB Function  TreatAsAtomicUnit=on
  myMux Fun2 : MATLAB Function  TreatAsAtomicUnit=on
  myMux Fun3 : MATLAB Function  TreatAsAtomicUnit=on
  myMux Fun4 : MATLAB Function  Commented=on  TreatAsAtomicUnit=on
  myMux Fun5 : MATLAB Function  Commented=on  TreatAsAtomicUnit=on
  myMux Fun6 : MATLAB Function  Commented=on  TreatAsAtomicUnit=on
  h_c : Outport
  phi_c : Outport  Port=2
  ISR Loc : Outport  Port=3
  "Puav " : Outport  Port=4
  wires:
  Data Type Conversion8/1 -> Log 1 navsupport.c [updated 5.1.16]1/1
  From50/1 -> myMux Fun5/1(u1)
  From52/1 -> myMux Fun5/2(u2)
  From51/1 -> myMux Fun5/3(u3)
  myMux Fun5/1(y) -> Data Type Conversion8/1
  Data Type Conversion7/1 -> myMux Fun4/3(u3)
  Data Type Conversion4/1 -> myMux Fun4/2(u2)
  Data Type Conversion3/1 -> myMux Fun4/1(u1)
  From49/1 -> Data Type Conversion7/1
  From36/1 -> Data Type Conversion3/1
  From29/1 -> Data Type Conversion4/1
  myMux Fun4/1(y) -> Data Type Conversion2/1
  Data Type Conversion2/1 -> Log 2 navsupport.c [updated 5.1.16]1/1
  [GSAlt] -> myMux Fun3/2(u2)
  Geod2LTP/1 -> Demux2/1
  Demux2/2 -> Terminator/1
  Demux2/1 -> myMux Fun3/1(u1)
  myMux Fun3/1(y) -> ISR Loc/1
  [GSRIn] -> Geod2LTP/2
  [GSLatLon] -> Geod2LTP/1
  Demux1/3 -> Geod2LTP/5
  Demux1/2 -> Geod2LTP/4
  Demux1/1 -> Geod2LTP/3
  Data Type Conversion1/1 -> Diagnoistics Set navsupport.c [updated 5.1.16]1/1
  [DFloat3] -> myMux Fun2/3(u3)
  [DFloat1] -> myMux Fun2/1(u1)
  [DFloat2] -> myMux Fun2/2(u2)
  ISR Scale/1 -> Minimum Turn Radius/2(Scale Factor)
  U_c/1 -> Minimum Turn Radius/1(U_c)
  ISR Location/1 -> Demux1/1, Circle Navigation/4(ISR Location)
  [Vxyz2D] -> Circle Navigation/8(Vxyz)
  T*(m)_1/1 -> Circle Navigation/7(T*)
  [V_g_norm] -> Circle Navigation/6(|V_g|)
  Minimum Turn Radius/1(R) -> Circle Navigation/5(R)
  [GSRIn] -> Circle Navigation/3(GS R)
  [GSLatLon] -> Circle Navigation/2(GS LatLon)
  Circle Navigation/5(ToWP) -> [tw_CI]
  Circle Navigation/4(FromWP) -> [fw_CI]
  Circle Navigation/3(Dist2Go) -> [dg_CI]
  Circle Navigation/1(L2_vec) -> [L2v_CI]
  Circle Navigation/2(h_c) -> [hc_CI]
  [Puav2D] -> Circle Navigation/1(Puav)
  Integer Delay1/1 -> [tw_WP]
  Integer Delay/1 -> [fw_WP]
  Line Segment/5(ToWP) -> [tw_LS]
  Normal WP Navigation/5(ToWP) -> Integer Delay1/1
  RTB/Follow Mobile Navigation/5(ToWP) -> [tw_RTB]
  Line Segment/4(FromWP) -> [fw_LS]
  Normal WP Navigation/4(FromWP) -> Integer Delay/1
  RTB/Follow Mobile Navigation/4(FromWP) -> [fw_RTB]
  Line Segment/3(Dist2Go) -> [dg_LS]
  Normal WP Navigation/3(Dist2Go) -> [dg_WP]
  RTB/Follow Mobile Navigation/3(Dist2Go) -> [dg_RTB]
  Merge3/1 -> [fromWp]
  Merge4/1 -> [toWp]
  Merge2/1 -> [dist2Go], To Workspace/1
  [tw_RTB] -> Merge4/1
  [tw_WP] -> Merge4/2
  [tw_LS] -> Merge4/3
  [tw_CI] -> Merge4/4
  [fw_RTB] -> Merge3/1
  [fw_WP] -> Merge3/2
  [fw_LS] -> Merge3/3
  [fw_CI] -> Merge3/4
  [dg_RTB] -> Merge2/1
  [dg_WP] -> Merge2/2
  [dg_LS] -> Merge2/3
  [dg_CI] -> Merge2/4
  L2+/2(eta) -> [totDist], Goto24/1, To Workspace1/1
  Data Type Conversion6/1 -> myMux Fun1/4(u4)
  Data Type Conversion5/1 -> myMux Fun1/3(u3)
  [toWp] -> Data Type Conversion6/1
  [fromWp] -> Data Type Conversion5/1
  [dist2Go] -> myMux Fun1/2(u2)
  [totDist] -> myMux Fun1/1(u1)
  myMux Fun1/1(y) -> getXYZ() navsupport.c [updated 5.1.16]/1
  Vxyz/1 -> Zero out Z1/1(Pin)
  Get 2D Groundspeed/1(|V_g|) -> [V_g_norm]
  [Vxyz2D] -> L2+/3(Vxyz)
  [V_g_norm] -> L2+/1(|V_g|)
  L2+/1(phi_c) -> phi_c/1
  T*(m)/1 -> L2+/4(T*(m))
  NavMode/1 -> Determine Overall Nav by the Nav Mode/1, Goto43/1, To Workspace4/1
  Merge/1 -> L2+/2(L2_vec), Goto23/1, To Workspace2/1
  Recent Enable/1(WPEnable) -> [wpEnable]
  Recent Enable/2("GS, Lat Lon") -> [GSLatLon], Demux3/1
  Recent Enable/3(GS R_in) -> [GSRIn], Demux/1
  RTB/1 -> Determine Overall Nav by the Nav Mode/2
  Follow Mobile?/1 -> RTB/Follow Mobile Navigation/2(Follow Mobile?)
  MidLvl h_c/1 -> RTB/Follow Mobile Navigation/3(MidLvl h_c)
  Mobile Location/1 -> RTB/Follow Mobile Navigation/1(Mobile Location)
  Zero out Z1/1(P) -> Get 2D Groundspeed/1(Vxyz), [Vxyz2D]
  Puav/1 -> "Puav "/1, Zero out Z2/1(Pin)
  [GSRIn] -> Normal WP Navigation/3(GS_R_in)
  [GSLatLon] -> Normal WP Navigation/2(GS_LatLon)
  [wpEnable] -> Normal WP Navigation/1(wpEnable)
  [V_g_norm] -> Normal WP Navigation/4(|V_g|)
  T*(m)_2/1 -> Normal WP Navigation/5(T*)
  [Puav2D] -> Normal WP Navigation/6(Puav)
  TurnLeadTime/1 -> Normal WP Navigation/7(TurnLeadTime)
  Max WP Idx/1 -> Normal WP Navigation/8(MaxWp)
  [GSLatLon] -> RTB/Follow Mobile Navigation/4(GS LatLon)
  [GSRIn] -> RTB/Follow Mobile Navigation/5(GS R)
  Zero out Z2/1(P) -> [Puav2D]
  [Puav2D] -> RTB/Follow Mobile Navigation/6(Puav)
  Merge1/1 -> h_c/1
  RTB/Follow Mobile Navigation/1(L2_vec) -> [L2v_RTB]
  RTB/Follow Mobile Navigation/2(h_c) -> [hc_RTB]
  Normal WP Navigation/1(L2_vec) -> [L2v_WP]
  Normal WP Navigation/2(h_c) -> [hc_WP]
  Line Segment/1(L2_vec) -> [L2v_LS]
  Line Segment/2(h_c) -> [hc_LS]
  [L2v_RTB] -> Merge/1
  [L2v_WP] -> Merge/2
  [L2v_LS] -> Merge/3
  [L2v_CI] -> Merge/4
  [hc_RTB] -> Merge1/1
  [hc_WP] -> Merge1/2
  [hc_LS] -> Merge1/3
  [hc_CI] -> Merge1/4
  [Puav2D] -> Line Segment/1(Puav)
  MidLvl h_c_1/1 -> Line Segment/2(MidLvl h_c)
  isApManual?/1 -> Logical Operator/1
  Logical Operator1/1 -> Recent Enable/1(WP Fly)
  Logical Operator/1 -> Logical Operator1/2
  WPFly/1 -> Logical Operator1/1
  myMux Fun2/1(y) -> Data Type Conversion1/1
  From54/1 -> Terminator1/1
  From53/1 -> Terminator2/1
  Demux/1 -> [DFloat1]
  Demux/2 -> [DFloat2]
  Demux3/1 -> Terminator4/1, Goto20/1
  Demux3/2 -> Terminator3/1, Goto21/1
  From57/1 -> Goto17/1
  Demux/3 -> [DFloat3]
  Recent Enable/4(GS Alt (m)) -> Terminator5/1, Goto19/1, [GSAlt]
  From58/1 -> myMux Fun6/3(u3)
  From56/1 -> myMux Fun6/1(u1)
  From55/1 -> myMux Fun6/2(u2)
  myMux Fun6/1(y) -> Data Type Conversion9/1
  Data Type Conversion9/1 -> Log 2 navsupport.c [updated 5.1.16]2/1
  Determine Overall Nav by the Nav Mode/1 -> RTB/Follow Mobile Navigation/Action
  Determine Overall Nav by the Nav Mode/2 -> Normal WP Navigation/Action
  Determine Overall Nav by the Nav Mode/3 -> Line Segment/Action
  Determine Overall Nav by the Nav Mode/4 -> Circle Navigation/Action

== system AUAV_V3_TestSensors/Position_and_Attitude_Filter/Attitude Complimentary Filter COG/3D Filter ==
  In1 : Inport
  Data Type Conversion1 : DataTypeConversion  OutDataTypeStr=single
  Data Type Conversion2 : DataTypeConversion  OutDataTypeStr=double
  Demux : Demux  Outputs=3
  Filter1 : Subsystem  mask(DiscretizedZeroPole){Zeros=zval, Poles=pval, Gain=kval, AbsTol=auto, SampleTime=TSample, method=tustin, Wc=1}
      mask prompts: Zeros "Zeros (enter in s-main:)"; Poles "Poles (enter in s-domain:)"; Gain "Gain (enter in s-domain:)"; AbsTol "Absolute tolerance:"; SampleTime "Sample time:"; Wc "Critical Frequency (Hz):"
      mask help: Continuous mask uses c2d to transform parameters onto the Discrete Zero-Pole block inside.
      mask init: same as AUAV_V3_TestSensors/Barometer_Driver/Baro Altimeter/Initial Baro Bias/Low Pass8
      mask TypeOptions method: zoh | foh | tustin | prewarp | matched
      mask Callback method: hidecrit
      mask Display:
      | droots(zeross,poless,gainss)
      | text( 0.5, 1.0, method, 'verticalAlignment','top')
  Filter2 : Subsystem  mask(DiscretizedZeroPole){Zeros=zval, Poles=pval, Gain=kval, AbsTol=auto, SampleTime=TSample, method=tustin, Wc=1}
      mask prompts: Zeros "Zeros (enter in s-main:)"; Poles "Poles (enter in s-domain:)"; Gain "Gain (enter in s-domain:)"; AbsTol "Absolute tolerance:"; SampleTime "Sample time:"; Wc "Critical Frequency (Hz):"
      mask help: Continuous mask uses c2d to transform parameters onto the Discrete Zero-Pole block inside.
      mask init: same as AUAV_V3_TestSensors/Barometer_Driver/Baro Altimeter/Initial Baro Bias/Low Pass8
      mask TypeOptions method: zoh | foh | tustin | prewarp | matched
      mask Callback method: hidecrit
      mask Display:
      | droots(zeross,poless,gainss)
      | text( 0.5, 1.0, method, 'verticalAlignment','top')
  Filter3 : Subsystem  mask(DiscretizedZeroPole){Zeros=zval, Poles=pval, Gain=kval, AbsTol=auto, SampleTime=TSample, method=tustin, Wc=1}
      mask prompts: Zeros "Zeros (enter in s-main:)"; Poles "Poles (enter in s-domain:)"; Gain "Gain (enter in s-domain:)"; AbsTol "Absolute tolerance:"; SampleTime "Sample time:"; Wc "Critical Frequency (Hz):"
      mask help: Continuous mask uses c2d to transform parameters onto the Discrete Zero-Pole block inside.
      mask init: same as AUAV_V3_TestSensors/Barometer_Driver/Baro Altimeter/Initial Baro Bias/Low Pass8
      mask TypeOptions method: zoh | foh | tustin | prewarp | matched
      mask Callback method: hidecrit
      mask Display:
      | droots(zeross,poless,gainss)
      | text( 0.5, 1.0, method, 'verticalAlignment','top')
  myMux Fun1 : MATLAB Function  TreatAsAtomicUnit=on
  Out1 : Outport
  wires:
  myMux Fun1/1(y) -> Data Type Conversion1/1
  In1/1 -> Data Type Conversion2/1
  Filter3/1(Out1) -> myMux Fun1/3(u3)
  Filter2/1(Out1) -> myMux Fun1/2(u2)
  Filter1/1(Out1) -> myMux Fun1/1(u1)
  Demux/3 -> Filter3/1(In1)
  Demux/2 -> Filter2/1(In1)
  Demux/1 -> Filter1/1(In1)
  Data Type Conversion2/1 -> Demux/1
  Data Type Conversion1/1 -> Out1/1

== system AUAV_V3_TestSensors/Position_and_Attitude_Filter/Attitude Complimentary Filter COG/Deriv  ==
  y : Inport
  Gain2 : Gain  Gain=[ 1/(5*apSampleTime) ]
  Integer Delay1 : Delay  DelayLength=5  InitialCondition=double(U_comm)  InputProcessing=Inherited  SampleTime=apSampleTime
  Sum5 : Sum  Inputs=-+|
  ydot : Outport
  wires:
  Sum5/1 -> Gain2/1
  Integer Delay1/1 -> Sum5/1
  y/1 -> Sum5/2, Integer Delay1/1
  Gain2/1 -> ydot/1

== system AUAV_V3_TestSensors/Position_and_Attitude_Filter/Attitude Complimentary Filter COG/Normalize Vector1 ==
  Vector : Inport
  Divide : Product  Inputs=*/
  Norm : Subsystem  AncestorBlock=SLUGS_Library/Navigation/Norm
  Zero Bound : Saturate  UpperLimit=inf  LowerLimit=0.001
  Normalized : Outport
  wires:
  Divide/1 -> Normalized/1
  Zero Bound/1 -> Divide/2
  Norm/1(Norm) -> Zero Bound/1
  Vector/1 -> Divide/1, Norm/1(Vector)

== system AUAV_V3_TestSensors/Position_and_Attitude_Filter/Attitude Complimentary Filter COG/Normalize Vector2 ==
  Vector : Inport
  Divide : Product  Inputs=*/
  Norm : Subsystem  AncestorBlock=SLUGS_Library/Navigation/Norm
  Zero Bound : Saturate  UpperLimit=inf  LowerLimit=0.001
  Normalized : Outport
  wires:
  Vector/1 -> Norm/1(Vector), Divide/1
  Norm/1(Norm) -> Zero Bound/1
  Zero Bound/1 -> Divide/2
  Divide/1 -> Normalized/1
